simulink model "CartesianControlSim"  (R2025b)
settings: Solver=VariableStepAuto  StartTime=0.0  StopTime=5  RelTol=1e-3
libraries: roblocks x1, matrix_library x1
settings Model: Creator=ckitt  LastModifiedBy=Jaxba

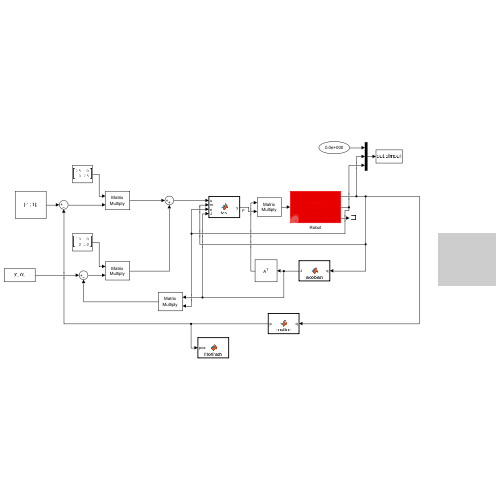
[thumbnail: Simulink's stored preview of the top-level diagram]
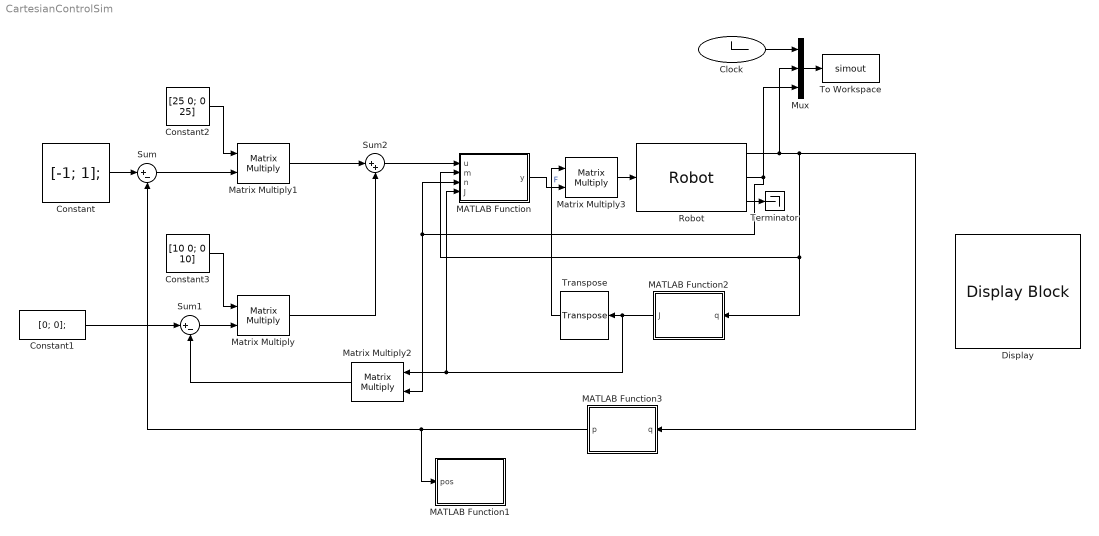
== system CartesianControlSim ==
  Clock : Clock
  Constant : Constant  Value=[-1; 1];
  Constant1 : Constant  Value=[0; 0];
  Constant2 : Constant  Value=[25 0; 0 25]
  Constant3 : Constant  Value=[10 0; 0 10]
  Display : DisplayBlock  LabelPosition=Hide  Transparency=1  GridColor=[0.502, 0.502, 0.502]
  MATLAB Function : MATLAB Function  TreatAsAtomicUnit=on
  MATLAB Function1 : MATLAB Function  TreatAsAtomicUnit=on
  MATLAB Function2 : MATLAB Function  TreatAsAtomicUnit=on
  MATLAB Function3 : MATLAB Function  TreatAsAtomicUnit=on
  Matrix Multiply{,1..3} (4 alike) : Product  Multiplication=Matrix(*)
  Mux : Mux  Inputs=3
  Robot : roblocks/Robot  robot=SCURRbot  q0=[0 pi/2]
      link override Integrator1: InitialCondition=q0
  Sum : Sum  Inputs=|+-
  Sum1 : Sum  Inputs=|+-
  Sum2 : Sum  Inputs=|++
  Terminator : Terminator
  To Workspace : ToWorkspace  VariableName=simout  SampleTime=-1
  Transpose : matrix_library/Transpose
  wires:
  Robot/3 -> Terminator/1
  Clock/1 -> Mux/1
  Mux/1 -> To Workspace/1
  Constant/1 -> Sum/1
  Constant1/1 -> Sum1/1
  Robot/2 -> Matrix Multiply2/2, MATLAB Function/3(n), Mux/3
  Sum1/1 -> Matrix Multiply/2
  Constant3/1 -> Matrix Multiply/1
  Sum/1 -> Matrix Multiply1/2
  Constant2/1 -> Matrix Multiply1/1
  Matrix Multiply1/1 -> Sum2/1
  Matrix Multiply/1 -> Sum2/2
  Sum2/1 -> MATLAB Function/1(u)
  Robot/1 -> Mux/2, MATLAB Function3/1(q), MATLAB Function2/1(q), MATLAB Function/2(m)
  MATLAB Function2/1(J) -> MATLAB Function/4(J), Matrix Multiply2/1, Transpose/1
  MATLAB Function3/1(p) -> MATLAB Function1/1(pos), Sum/2
  Matrix Multiply2/1 -> Sum1/2
  Matrix Multiply3/1 -> Robot/1
  MATLAB Function/1(y) -> Matrix Multiply3/2  "F"
  Transpose/1 -> Matrix Multiply3/1

== matlab function CartesianControlSim/MATLAB Function1 ==
  data: pos input
function PlotPath(pos)

% pos is [x; y]

persistent hFig hAx hTrail initialized

if isempty(initialized)
    % Create figure on first call
    hFig = figure(1001); clf;
    hAx = axes('Parent', hFig);
    hold(hAx, 'on');
    grid(hAx, 'on');
    axis(hAx, [-2 2 -2 2]);
    xlabel(hAx, 'X'); ylabel(hAx, 'Y');
    title(hAx, 'End-Effector Path Visualization');

    % Initialize trail plot
    hTrail = plot(hAx, pos(1), pos(2), 'b.-', 'LineWidth', 2);

    initialized = true;
end

% Append new point to the trail
xdata = get(hTrail, 'XData');
ydata = get(hTrail, 'YData');

set(hTrail, 'XData', [xdata pos(1)], ...
            'YData', [ydata pos(2)]);

drawnow limitrate
end

== matlab function CartesianControlSim/MATLAB Function ==
  data: u input; y output; m input; n input; J input
function y = fcn(u, m, n, J)

m1 = 3; m2 = 3; B1 = 3; B2 = 3;

m11 = m2+2*m2*cos(m(2))+(m1+m2);
m12 = m2+m2*cos(m(2));
m21 = m2+m2*cos(m(2));
m22 = m2;
M = [m11 m12; m21 m22];

V = [-m2*sin(m(2))*(n(2)^2) - 2*m2*sin(m(2))*n(1)*n(2); 
     m2*sin(m(2))*(n(1)^2)];

F = [B1*n(1); B2*n(2)];

Jinv = inv(J);
JinvT = Jinv';

Jdot11 = -cos(m(1))*n(1) - cos(m(1)+m(2))*(n(1)+n(2));
Jdot12 = -cos(m(1)+m(2)) * (n(1)+n(2));

Jdot21 = -sin(m(1))*n(1) - sin(m(1)+m(2)) * (n(1)+n(2));
Jdot22 = -sin(m(1)+m(2)) * (n(1)+n(2));

Jdot = [Jdot11 Jdot12;
        Jdot21 Jdot22];

Mx = JinvT * M * Jinv;

Vx = JinvT * ( V - M * (Jinv * (Jdot * n)) );

Fx = JinvT * F;


y = Mx*(u + (Jinv * (Jdot * n))) + Vx + Fx;
end

== matlab function CartesianControlSim/MATLAB Function2 ==
  data: q input; J output
function J = jacobian(q)

% 2x2 Jacobian for planar 2R arm
J11 = sin(q(1)) - sin(q(1)+q(2));
J12 = sin(q(1)+q(2));

J21 =  cos(q(1)) + cos(q(1)+q(2));
J22 =  cos(q(1)+q(2));

J = [J11 J12;
     J21 J22];
end

== matlab function CartesianControlSim/MATLAB Function3 ==
  data: q input; p output
function p = position(q)

% Forward kinematics
x = cos(q(1)) + cos(q(1) + q(2));
y = sin(q(1)) + sin(q(1) + q(2));

p = [x; y];
end
